simulink model "LQR_simulink"  (Simulink 9.3)
settings: Solver=ode3  StartTime=0.0  StopTime=3  FixedStep=T  RelTol=1e-3  EnableMultiTasking=on
values from neighbouring files (symbols this model uses):
  A = An    [Main_Vertical_Motion_Control.m]    (also in Main_for_DOCandDODR.m; System_model.m = A(2:end,2:end))
  Ar = Arn    [Main_Vertical_Motion_Control.m]    (also in Main_for_DOCandDODR.m; System_model.m = [0])
  B = Bn    [Main_Vertical_Motion_Control.m]    (also in Main_for_DOCandDODR.m; System_model.m = B(2:end,:))
  Br = Brn    [Main_Vertical_Motion_Control.m]    (also in Main_for_DOCandDODR.m; System_model.m = [2/(ms+4*mw)*ones(1,2)])
  T = 0.001    [Main_Vertical_Motion_Control.m]    (also in Main_for_DOCandDODR.m)
  xf = xfnend    [Main_Vertical_Motion_Control.m]    (also in Main_for_DOCandDODR.m)
  xfr = xfrnend    [Main_Vertical_Motion_Control.m]    (also in Main_for_DOCandDODR.m)
  xi = xin    [Main_Vertical_Motion_Control.m]    (also in Main_for_DOCandDODR.m)
  xir = xirn    (= 0.5)    [Main_Vertical_Motion_Control.m]    (also in Main_for_DOCandDODR.m)
undefined symbols (not defined in the file or in its folder): Kgain, Kgain_r
settings Model: Creator=JSPark  LastModifiedBy=jspark
settings OptimizationCC: ExpressionDepthLimit=2147483647
settings DebuggingCC: SolverPrmCheckMsg=warning  StateNameClashWarn=warning

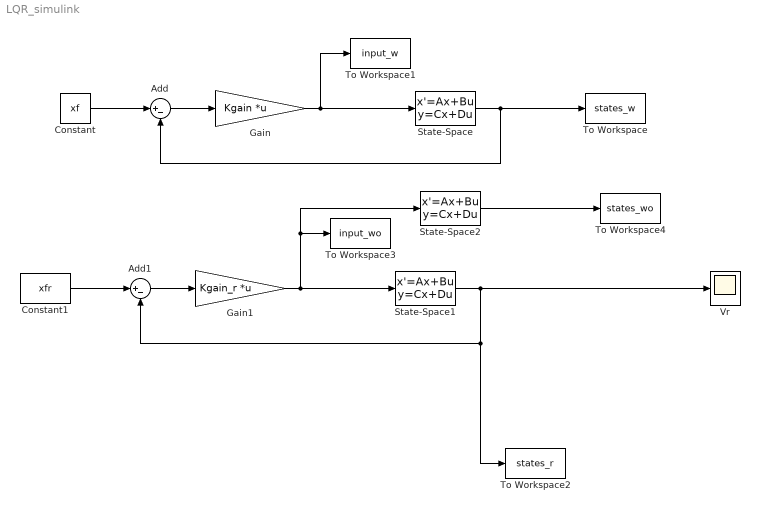
== system LQR_simulink ==
  Add : Sum  Inputs=|+-  SampleTime=T
  Add1 : Sum  Inputs=|+-  SampleTime=T
  Constant : Constant  Value=xf  SampleTime=T
  Constant1 : Constant  Value=xfr  SampleTime=T
  Gain : Gain  Gain=Kgain  Multiplication=Matrix(K*u)  SampleTime=T
  Gain1 : Gain  Gain=Kgain_r  Multiplication=Matrix(K*u)  SampleTime=T
  State-Space : StateSpace  A=A  B=B  C=eye(length(A))  D=zeros(length(A),2)  InitialCondition=xi
  State-Space1 : StateSpace  A=Ar  B=Br  C=eye(length(Ar))  D=zeros(length(Ar),2)  InitialCondition=xir
  State-Space2 : StateSpace  A=A  B=B  C=eye(length(A))  D=zeros(length(A),2)  InitialCondition=xi
  To Workspace : ToWorkspace  VariableName=states_w  SaveFormat=Structure  SampleTime=T
  To Workspace1 : ToWorkspace  VariableName=input_w  SaveFormat=Structure  SampleTime=T
  To Workspace2 : ToWorkspace  VariableName=states_r  SaveFormat=Structure  SampleTime=T
  To Workspace3 : ToWorkspace  VariableName=input_wo  SaveFormat=Structure  SampleTime=T
  To Workspace4 : ToWorkspace  VariableName=states_wo  SaveFormat=Structure  SampleTime=T
  Vr : Scope
  wires:
  State-Space/1 -> Add/2, To Workspace/1
  Add/1 -> Gain/1
  Constant/1 -> Add/1
  Gain/1 -> To Workspace1/1, State-Space/1
  Add1/1 -> Gain1/1
  Gain1/1 -> State-Space2/1, To Workspace3/1, State-Space1/1
  Constant1/1 -> Add1/1
  State-Space1/1 -> Vr/1, Add1/2, To Workspace2/1
  State-Space2/1 -> To Workspace4/1
